simulink model "MMMS_v2_dynamics"  (R2024b)
settings: Solver=VariableStepAuto  StartTime=0.0  StopTime=60  FixedStep=0.001  RelTol=1e-3
InitFcn:
  | %rho_0t=[0.29;0.29;0.29]; %m
  | %V_0t=[-0.001;-0.001;0];%[-0.0005;-0.0005;0];
  | %w_t=[0;0;-0.002];
  | 
  | 
  | %rho_0t=[0.3;0.3;0.2]; %m
  | %V_0t=[-0.001;-0.001;0];%[-0.0005;-0.0005;0];
  | %w_t=[0;0;-0.001];
values from neighbouring files (symbols this model uses):
  Dt = 0.1    [main_EKF.m]
  Fake_Manip_grad = -0.2.*eye(7)    [Initiate_FQ.m]
  g_cm = zeros(4,4,n)    [Initiate_KUKA_inv.m]    (also in Main_MMMS.m; test_KUKA_elements.m)
  g_It00 = [eye(3) rho_It;0 0 0 1]    [main_EKF.m]
  iota0 = eye(6,6)    [Initiate_KUKA_inv.m]    (also in Main_MMMS.m; test_KUKA_elements.m)
  K_d = 10*[1.3*eye(3) zeros(3);zeros(3) 0.8*eye(3)]    [Initiate_FQ.m]    (also in Initiate_KUKA_inv.m = 5*[0.7*eye(3) zeros(3);zeros(3) 0.5*eye(3)]; MMMS_Initiate_FQ.m; Main_MMMS.m = 5*[0.7*eye(3) zeros(3);zeros(3) 0.5*eye(3)]; test_KUKA_elements.m = 50*[0.7*eye(3) zeros(3);zeros(3) 0.5*eye(3)])
  K_i = 5*[0.1*eye(3) zeros(3);zeros(3) 0.01*eye(3)]    [Initiate_FQ.m]    (also in Initiate_KUKA_inv.m = 5*[0.01*eye(3) zeros(3);zeros(3) 0.001*eye(3)]; MMMS_Initiate_FQ.m; Main_MMMS.m = 5*[0.01*eye(3) zeros(3);zeros(3) 0.001*eye(3)]; test_KUKA_elements.m = 50*[0.01*eye(3) zeros(3);zeros(3) 0.001*eye(3)])
  K_p = 100*[0.1 0 0 0 0 0;0 0.1 0 0 0 0; 0 0 0.1 0 0 0; 0 0 0 0.01 0 0 ... (first row only)    [Initiate_FQ.m]    (also in Initiate_KUKA_inv.m = 5*[0.1 0 0 0 0 0;0 0.1 0 0 0 0; 0 0 0.1 0 0 0; 0 0 0 0.01 0 ; MMMS_Initiate_FQ.m; Main_MMMS.m = 5*[0.1 0 0 0 0 0;0 0.1 0 0 0 0; 0 0 0.1 0 0 0; 0 0 0 0.01 0 ; test_KUKA_elements.m = 50*[0.1 0 0 0 0 0;0 0.1 0 0 0 0; 0 0 0.1 0 0 0; 0 0 0 0.01 0)
  K_w = 200*eye(7)    [Initiate_FQ.m]    (also in MMMS_Initiate_FQ.m)
  K_wd = 2*eye(7)    [Initiate_FQ.m]    (also in MMMS_Initiate_FQ.m)
  m = randn(s,total_time_steps,6)*chol(R)    [main_EKF.m]
  M0 = M_temp.M0.data(:,:,1)    [Initiate_FQ.m]    (also in MMMS_Initiate_FQ.m; test_KUKA_elements.m)
  m0 = robot.Bodies{1,n+1}.Mass    [Initiate_KUKA_inv.m]    (also in Main_MMMS.m; test_KUKA_elements.m)
  m0_frak = diag_M(1:6,1:6)    [Initiate_KUKA_inv.m]    (also in Main_MMMS.m; make_uncertain.m = diag_M_unc(1:6,1:6); test_KUKA_elements.m)
  M0m = M_temp.M0m.data(:,:,1)    [Initiate_FQ.m]    (also in MMMS_Initiate_FQ.m; test_KUKA_elements.m)
  m_diag = diag_M(7:end,7:end)    [Initiate_KUKA_inv.m]    (also in Main_MMMS.m; make_uncertain.m = diag_M_unc(7:end,7:end); test_KUKA_elements.m)
  M_t = (((Adjoint(g_It))'\M_t_body)/(Adjoint(g_It)))    [Initiate_FQ.m]    (also in Initiate_KUKA_inv.m = [eye(3)*mt zeros(3); zeros(3) eye(3)*80]; MMMS_Initiate_FQ.m; Main_MMMS.m = [eye(3)*mt zeros(3); zeros(3) eye(3)*80]; test_KUKA_elements.m = [eye(3)*mt zeros(3); zeros(3) eye(3)*80])
  M_t_body = [eye(3)*mt zeros(3); zeros(3) eye(3)*0.416667]    [Initiate_FQ.m]    (also in MMMS_Initiate_FQ.m)
  mm = zeros(1,n)    [Initiate_KUKA_inv.m]    (also in Main_MMMS.m; test_KUKA_elements.m)
  mu = P0    [Initiate_FQ.m]    (also in Initiate_KUKA_inv.m = zeros(6,1); MMMS_Initiate_FQ.m; Main_MMMS.m = zeros(6,1); make_uncertain.m = P0_unc)
  mu_t = inv((Adjoint(g_It))')*M_t_body*[V_It;w_t]    [Initiate_FQ.m]    (also in Initiate_KUKA_inv.m = M_t*[V_0t;w_t]; MMMS_Initiate_FQ.m; Main_MMMS.m = M_t*[V_0t;w_t]; make_uncertain.m = inv((Adjoint(g_It))')*M_t_body_unc*[V_It;w_t])
  noise_st = 0.000005    (= 5e-06)    [main_EKF.m]
  q_dot_m = [0;0;0;0;0;0;0]    [Initiate_FQ.m]    (also in Initiate_KUKA_inv.m; MMMS_Initiate_FQ.m; Main_MMMS.m; test_KUKA_elements.m = [0])
  q_m = [0.2;1.2;0.3;2.5;0.5;1.5;0.6]    [Initiate_FQ.m]    (also in Initiate_KUKA_inv.m = [0;0;0;0;0;0;0]; MMMS_Initiate_FQ.m = [0.2;0.2;0.3;0.5;0.5;0.5;0.6]; Main_MMMS.m = [0;0;0;0;0;0;0]; test_KUKA_elements.m = [0.2;1.2;0.3;1.8;0.5;1.3;0.6])
  rho_It = [0;0;1.7]    [Initiate_FQ.m]    (also in MMMS_Initiate_FQ.m)
  s = RandStream.create('mrg32k3a','NumStreams',1)    [main_EKF.m]
  sc_size = 1    [Initiate_KUKA_inv.m]    (also in Main_MMMS.m; test_KUKA_elements.m)
  V_It = [0.0005;0.0005;0]    [Initiate_FQ.m]    (also in MMMS_Initiate_FQ.m = [0.001;0.001;0])
  Xi_m_matrix = zeros(6*n,n)    [Initiate_KUKA_inv.m]    (also in Main_MMMS.m)
undefined symbols (not defined in the file or in its folder): g_cm0, I0, Im, Mm, X, Xi_m, Y, Z
libraries: nesl_utility x314, sm_lib x231, robotcorelib x30, simulink x12
(part 4 of 14)

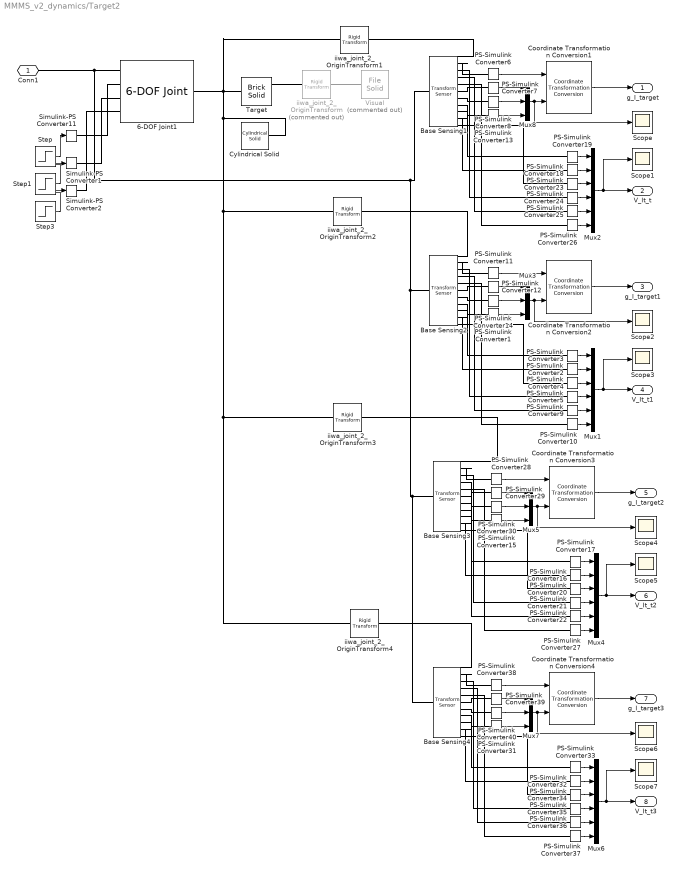
== system MMMS_v2_dynamics/Target2 ==
  6-DOF Joint1 : sm_lib/Joints/6-DOF Joint  JointMode=Normal  CompositeWrenchDir=FollowerOnBase  CompositeWrenchFrame=BaseFrame  SenseConstraintForce=off  SenseConstraintTorque=off  SenseTotalForce=off  SenseTotalTorque=off  PxPositionTargetSpecify=on  PxPositionTargetPriority=High  PxPositionTargetValue=rho_It(1)  PxPositionTargetValueUnits=m  PxVelocityTargetSpecify=on  PxVelocityTargetPriority=High  PxVelocityTargetValue=V_It(1)  PxVelocityTargetValueUnits=m/s  PxEquilibriumPosition=0  PxEquilibriumPositionUnits=m  PxSpringStiffness=0  PxSpringStiffnessUnits=N/m  PxDampingCoefficient=0  PxDampingCoefficientUnits=N/(m/s)  PxLowerLimitSpecify=off  PxLowerLimitBound=-1  PxLowerLimitBoundUnits=m  PxLowerLimitStiffness=1e6  PxLowerLimitStiffnessUnits=N/m  PxLowerLimitDamping=1e3  PxLowerLimitDampingUnits=N/(m/s)  PxLowerLimitTransitionRegionWidth=1e-4  PxLowerLimitTransitionRegionWidthUnits=m  PxUpperLimitSpecify=off  PxUpperLimitBound=1  PxUpperLimitBoundUnits=m  PxUpperLimitStiffness=1e6  PxUpperLimitStiffnessUnits=N/m  PxUpperLimitDamping=1e3  PxUpperLimitDampingUnits=N/(m/s)  PxUpperLimitTransitionRegionWidth=1e-4  PxUpperLimitTransitionRegionWidthUnits=m  PxTorqueActuationMode=InputTorque  PxMotionActuationMode=ComputedMotion  PxSensePosition=off  PxSenseVelocity=off  PxSenseAcceleration=off  PxSenseTorqueForce=off  PxSenseLowerLimitTorqueForce=off  PxSenseUpperLimitTorqueForce=off  PyPositionTargetSpecify=on  PyPositionTargetPriority=High  PyPositionTargetValue=rho_It(2)  PyPositionTargetValueUnits=m  PyVelocityTargetSpecify=on  PyVelocityTargetPriority=High  PyVelocityTargetValue=V_It(2)  PyVelocityTargetValueUnits=m/s  PyEquilibriumPosition=0  PyEquilibriumPositionUnits=m  PySpringStiffness=0  PySpringStiffnessUnits=N/m  PyDampingCoefficient=0  PyDampingCoefficientUnits=N/(m/s)  PyLowerLimitSpecify=off  PyLowerLimitBound=-1  PyLowerLimitBoundUnits=m  PyLowerLimitStiffness=1e6  PyLowerLimitStiffnessUnits=N/m  PyLowerLimitDamping=1e3  PyLowerLimitDampingUnits=N/(m/s)  PyLowerLimitTransitionRegionWidth=1e-4  PyLowerLimitTransitionRegionWidthUnits=m  PyUpperLimitSpecify=off  PyUpperLimitBound=1  PyUpperLimitBoundUnits=m  PyUpperLimitStiffness=1e6  PyUpperLimitStiffnessUnits=N/m  PyUpperLimitDamping=1e3  PyUpperLimitDampingUnits=N/(m/s)  PyUpperLimitTransitionRegionWidth=1e-4  PyUpperLimitTransitionRegionWidthUnits=m  PyTorqueActuationMode=InputTorque  PyMotionActuationMode=ComputedMotion  PySensePosition=off  PySenseVelocity=off  PySenseAcceleration=off  PySenseTorqueForce=off  PySenseLowerLimitTorqueForce=off  PySenseUpperLimitTorqueForce=off  PzPositionTargetSpecify=on  PzPositionTargetPriority=High  PzPositionTargetValue=rho_It(3)-0.1  PzPositionTargetValueUnits=m  PzVelocityTargetSpecify=on  PzVelocityTargetPriority=High  PzVelocityTargetValue=V_It(3)  PzVelocityTargetValueUnits=m/s  PzEquilibriumPosition=0  PzEquilibriumPositionUnits=m  PzSpringStiffness=0  PzSpringStiffnessUnits=N/m  PzDampingCoefficient=0  PzDampingCoefficientUnits=N/(m/s)  PzLowerLimitSpecify=off  PzLowerLimitBound=-1  PzLowerLimitBoundUnits=m  PzLowerLimitStiffness=1e6  PzLowerLimitStiffnessUnits=N/m  PzLowerLimitDamping=1e3  PzLowerLimitDampingUnits=N/(m/s)  PzLowerLimitTransitionRegionWidth=1e-4  PzLowerLimitTransitionRegionWidthUnits=m  PzUpperLimitSpecify=off  PzUpperLimitBound=1  PzUpperLimitBoundUnits=m  PzUpperLimitStiffness=1e6  PzUpperLimitStiffnessUnits=N/m  PzUpperLimitDamping=1e3  PzUpperLimitDampingUnits=N/(m/s)  PzUpperLimitTransitionRegionWidth=1e-4  PzUpperLimitTransitionRegionWidthUnits=m  PzTorqueActuationMode=InputTorque  PzMotionActuationMode=ComputedMotion  PzSensePosition=off  PzSenseVelocity=off  PzSenseAcceleration=off  PzSenseTorqueForce=off  PzSenseLowerLimitTorqueForce=off  PzSenseUpperLimitTorqueForce=off  SphPositionTargetSpecify=on  SphPositionTargetPriority=High  SphPositionTargetRotationMethod=RotationSequence  SphPositionTargetFollAlignAxisA=+X  SphPositionTargetBaseAlignAxisA=+Y  SphPositionTargetFollAlignAxisB=+Y  SphPositionTargetBaseAlignAxisB=+Z  SphPositionTargetRotationStandardAxis=+Z  SphPositionTargetRotationAngle=0.0  SphPositionTargetRotationAngleUnits=deg  SphPositionTargetRotationArbitraryAxis=[0 0 1]  SphPositionTargetRotationSequenceAxes=FollowerAxes  SphPositionTargetRotationSequence=XYZ  SphPositionTargetRotationSequenceAngles=[0 0 0]  SphPositionTargetRotationSequenceAnglesUnits=rad  SphPositionTargetRotationMatrix=[1 0 0; 0 1 0; 0 0 1]  SphPositionTargetQuaternion=[1 0 0 0]  SphVelocityTargetSpecify=on  SphVelocityTargetPriority=High  SphVelocityTargetValue=w_t  SphVelocityTargetValueUnits=rad/s  SphVelocityTargetInFollowerFrame=off  SphEqPosRotationMethod=None  SphEqPosFollAlignAxisA=+X  SphEqPosBaseAlignAxisA=+Y  SphEqPosFollAlignAxisB=+Y  SphEqPosBaseAlignAxisB=+Z  SphEqPosRotationStandardAxis=+Z  SphEqPosRotationAngle=0.0  SphEqPosRotationAngleUnits=deg  SphEqPosRotationArbitraryAxis=[0 0 1]  SphEqPosRotationSequenceAxes=FollowerAxes  SphEqPosRotationSequence=XYX  SphEqPosRotationSequenceAngles=[0 0 0]  SphEqPosRotationSequenceAnglesUnits=deg  SphEqPosRotationMatrix=[1 0 0; 0 1 0; 0 0 1]  SphEqPosQuaternion=[1 0 0 0]  SphSpringStiffness=0  SphSpringStiffnessUnits=N*m/deg  SphDampingCoefficient=0  SphDampingCoefficientUnits=N*m/(deg/s)  SphLowerLimitSpecify=off  SphLowerLimitBound=15  SphLowerLimitBoundUnits=deg  SphLowerLimitStiffness=1e4  SphLowerLimitStiffnessUnits=N*m/deg  SphLowerLimitDamping=10  SphLowerLimitDampingUnits=N*m/(deg/s)  SphLowerLimitTransitionRegionWidth=0.1  SphLowerLimitTransitionRegionWidthUnits=deg  SphUpperLimitSpecify=off  SphUpperLimitBound=45  SphUpperLimitBoundUnits=deg  SphUpperLimitStiffness=1e4  SphUpperLimitStiffnessUnits=N*m/deg  SphUpperLimitDamping=10  SphUpperLimitDampingUnits=N*m/(deg/s)  SphUpperLimitTransitionRegionWidth=0.1  SphUpperLimitTransitionRegionWidthUnits=deg  SphTorqueActuationMode=NoTorque  SphActuateTorqueX=off  SphActuateTorqueY=off  SphActuateTorqueZ=off  SphActuateTorque=off  SphActuationFrame=BaseFrame  SphSensePosition=off  SphSenseVelocityX=off  SphSenseVelocityY=off  SphSenseVelocityZ=off  SphSenseVelocity=off  SphSenseAccelerationX=off  SphSenseAccelerationY=off  SphSenseAccelerationZ=off  SphSenseAcceleration=off  SphSenseLowerLimitTorqueMag=off  SphSenseUpperLimitTorqueMag=off  SphSensingFrame=BaseFrame
  Base Sensing{1..4} (4 alike) : sm_lib/Frames and Transforms/Transform Sensor  MeasurementFrame=NonRotatingBase  RotationSequence=XYZ  SenseAngle=off  SenseAxis=off  SenseQ=off  SenseR=on  SenseRotationSequence=off  SenseOmegaX=on  SenseOmegaY=on  SenseOmegaZ=on  SenseOmega=off  SenseQDot=off  SenseRDot=off  SenseRotationSequenceDot=off  SenseAlphaX=off  SenseAlphaY=off  SenseAlphaZ=off  SenseAlpha=off  SenseQDDot=off  SenseRDDot=off  SenseX=on  SenseY=on  SenseZ=on  SenseXYZ=off  SenseRad=off  SenseAzim=off  SenseDist=off  SenseInc=off  SenseXDot=on  SenseYDot=on  SenseZDot=on  SenseXYZDot=off  SenseRadDot=off  SenseAzimDot=off  SenseDistDot=off  SenseIncDot=off  SenseXDDot=off  SenseYDDot=off  SenseZDDot=off  SenseXYZDDot=off  SenseRadDDot=off  SenseAzimDDot=off  SenseDistDDot=off  SenseIncDDot=off
  Coordinate Transformation Conversion{1..4} (4 alike) : robotcorelib/Coordinate Transformation Conversion  InputRepresentation=Rotation Matrix  InputEulerSequence=ZYX  ShowTrVecInputPort=on  OutputRepresentation=Homogeneous Transformation  OutputEulerSequence=ZYX  ShowTrVecOutputPort=on  SimulateUsing=Interpreted execution
  Cylindrical Solid : sm_lib/Body Elements/Cylindrical Solid  CylinderRadius=1  CylinderRadiusUnits=m  CylinderLength=0.001  CylinderLengthUnits=m  ExportEntireGeometry=off  InertiaType=CalculateFromGeometry  BasedOnType=Density  Density=0  DensityUnits=kg/m^3  Mass=1  MassUnits=kg  CenterOfMass=[0 0 0]  CenterOfMassUnits=m  MomentsOfInertia=[1 1 1]  MomentsOfInertiaUnits=kg*m^2  ProductsOfInertia=[0 0 0]  ProductsOfInertiaUnits=kg*m^2  GraphicType=FromGeometry  MarkerShape=Sphere  MarkerSize=10  GraphicVisPropType=SimpleVisualProperties  GraphicDiffuseColor=[1.0 0.0 0.0]  GraphicOpacity=0.4  GraphicSpecularColor=[0.5 0.5 0.5 1.0]  GraphicAmbientColor=[0.15 0.15 0.15 1.0]  GraphicEmissiveColor=[0.0 0.0 0.0 1.0]  GraphicShininess=75  DoExposeReferenceFrame=on  SerializedFrames=<Frames/>
  Mux{1..2,4,6} (4 alike) : Mux  Inputs=6
  Mux{3,5,7..8} (4 alike) : Mux  Inputs=3
  PS-Simulink Converter{1..40} (40 alike) : nesl_utility/PS-Simulink Converter  PhysicalDomain=network_engine_domain  SubClassName=ps_output  LeftPortType=input  RightPortType=output  PseudoPeriodic=off  Frequencies=[]  VectorFormat=1-D array  Unit=inherit  AffineConversion=off
  Scope{,1..7} (8 alike) : Scope
  Simulink-PS Converter1 : nesl_utility/Simulink-PS Converter  PhysicalDomain=network_engine_domain  SubClassName=ps_input  LeftPortType=input  RightPortType=output  PseudoPeriodic=off  Frequencies=[]  NoiseDistribution=none  NoiseParameters=[]  Unit=1  AffineConversion=off  FilteringAndDerivatives=provide  SimscapeFilterOrder=1  InputFilterTimeConstant=0.001  UdotUserProvided=0
  Simulink-PS Converter11 : nesl_utility/Simulink-PS Converter  PhysicalDomain=network_engine_domain  SubClassName=ps_input  LeftPortType=input  RightPortType=output  PseudoPeriodic=off  Frequencies=[]  NoiseDistribution=none  NoiseParameters=[]  Unit=1  AffineConversion=off  FilteringAndDerivatives=provide  SimscapeFilterOrder=1  InputFilterTimeConstant=0.001  UdotUserProvided=0
  Simulink-PS Converter2 : nesl_utility/Simulink-PS Converter  PhysicalDomain=network_engine_domain  SubClassName=ps_input  LeftPortType=input  RightPortType=output  PseudoPeriodic=off  Frequencies=[]  NoiseDistribution=none  NoiseParameters=[]  Unit=1  AffineConversion=off  FilteringAndDerivatives=provide  SimscapeFilterOrder=1  InputFilterTimeConstant=0.001  UdotUserProvided=0
  Step : Step  Time=50  After=-0.004  SampleTime=0
  Step1 : Step  Time=50  After=-0.004  SampleTime=0
  Step3 : Step  Time=50  After=-0.0002  SampleTime=0
  Target : sm_lib/Body Elements/Brick Solid  BrickDimensions=[0.5, 0.5, 0.5]  BrickDimensionsUnits=m  ExportEntireGeometry=on  InertiaType=Custom  BasedOnType=Mass  Density=1000  DensityUnits=kg/m^3  Mass=10  MassUnits=kg  CenterOfMass=[0 0 0]  CenterOfMassUnits=m  MomentsOfInertia=[M_t(4,4) M_t(5,5) M_t(6,6)]  MomentsOfInertiaUnits=kg*m^2  ProductsOfInertia=[0 0 0]  ProductsOfInertiaUnits=kg*m^2  GraphicType=None  MarkerShape=Sphere  MarkerSize=10  GraphicVisPropType=SimpleVisualProperties  GraphicDiffuseColor=[1.0 0.0 0.0]  GraphicOpacity=1.0  GraphicSpecularColor=[0.5 0.5 0.5 1.0]  GraphicAmbientColor=[0.15 0.15 0.15 1.0]  GraphicEmissiveColor=[0.0 0.0 0.0 1.0]  GraphicShininess=75  DoExposeReferenceFrame=on  SerializedFrames=<Frames><Frame><Id>Frame1</Id><Value><Name>F1</Name><Origin><Source>GeometricFeature</Source><FeatureName>-x -y -z point</FeatureName></Origin><PrimaryAxis><DefinedDirection>+Z</DefinedDirection><Source>ReferenceFrame</Source><SourceDirection>+Z</SourceDirection><FeatureName></FeatureName></PrimaryAxis><SecondaryAxis><DefinedDirection>+X</DefinedDirection><Source>ReferenceFrame</Source><SourceDirection>+X</SourceDirection><FeatureName></FeatureName></SecondaryAxis></Value></Frame></Frames>
  Visual : sm_lib/Body Elements/File Solid  Commented=on  ExtGeomFileName=Spacecrafts/CubeSatAssembly_wo_antennas.stl  UnitType=Custom  ExtGeomFileUnits=cm  StepReaderType=HEX  ExportConvexHullGeometry=off  InertiaType=Custom  BasedOnType=DensityFromFile  Density=1000  DensityUnits=kg/m^3  Mass=0  MassUnits=kg  CenterOfMass=[0, 0, 0]  CenterOfMassUnits=m  MomentsOfInertia=[0, 0, 0]  MomentsOfInertiaUnits=kg*m^2  ProductsOfInertia=[0, 0, 0]  ProductsOfInertiaUnits=kg*m^2  GraphicType=FromGeometry  MarkerShape=Sphere  MarkerSize=10  GraphicVisPropType=SimpleVisualProperties  GraphicDiffuseColor=[0.7 0.7 0.7]  GraphicOpacity=1  GraphicSpecularColor=[0.5 0.5 0.5 1.0]  GraphicAmbientColor=[0.15 0.15 0.15 1.0]  GraphicEmissiveColor=[0.0 0.0 0.0 1.0]  GraphicShininess=75  DoExposeReferenceFrame=on  SerializedFrames=<Frames/>
  iiwa_joint_2_OriginTransform : sm_lib/Frames and Transforms/Rigid Transform  Commented=on  RotationMethod=RotationSequence  FollAlignAxisA=+X  BaseAlignAxisA=+Y  FollAlignAxisB=+Y  BaseAlignAxisB=+Z  RotationStandardAxis=+Z  RotationAngle=0.0  RotationAngleUnits=deg  RotationArbitraryAxis=[0 0 1]  RotationSequenceAxes=FollowerAxes  RotationSequence=XYZ  RotationSequenceAngles=[0 0 0]  RotationSequenceAnglesUnits=rad  RotationMatrix=[1 0 0; 0 1 0; 0 0 1]  Quaternion=[1 0 0 0]  TranslationMethod=Cartesian  TranslationCartesianOffset=[-3.28, -4.43, 0.817]+[0.25, 0.25, 0.25]  TranslationCartesianOffsetUnits=m  TranslationStandardAxis=+Z  TranslationStandardOffset=0  TranslationStandardOffsetUnits=m  TranslationROffset=0  TranslationROffsetUnits=m  TranslationThetaOffset=0  TranslationThetaOffsetUnits=deg  TranslationZOffset=0  TranslationZOffsetUnits=m
  iiwa_joint_2_OriginTransform1 : sm_lib/Frames and Transforms/Rigid Transform  RotationMethod=RotationSequence  FollAlignAxisA=+X  BaseAlignAxisA=+Y  FollAlignAxisB=+Y  BaseAlignAxisB=+Z  RotationStandardAxis=+Z  RotationAngle=0.0  RotationAngleUnits=deg  RotationArbitraryAxis=[0 0 1]  RotationSequenceAxes=FollowerAxes  RotationSequence=XYZ  RotationSequenceAngles=[0 0 0]  RotationSequenceAnglesUnits=rad  RotationMatrix=[1 0 0; 0 1 0; 0 0 1]  Quaternion=[1 0 0 0]  TranslationMethod=Cartesian  TranslationCartesianOffset=[-1,0,0]  TranslationCartesianOffsetUnits=m  TranslationStandardAxis=+Z  TranslationStandardOffset=0  TranslationStandardOffsetUnits=m  TranslationROffset=0  TranslationROffsetUnits=m  TranslationThetaOffset=0  TranslationThetaOffsetUnits=deg  TranslationZOffset=0  TranslationZOffsetUnits=m
  iiwa_joint_2_OriginTransform2 : sm_lib/Frames and Transforms/Rigid Transform  RotationMethod=RotationSequence  FollAlignAxisA=+X  BaseAlignAxisA=+Y  FollAlignAxisB=+Y  BaseAlignAxisB=+Z  RotationStandardAxis=+Z  RotationAngle=0.0  RotationAngleUnits=deg  RotationArbitraryAxis=[0 0 1]  RotationSequenceAxes=FollowerAxes  RotationSequence=XYZ  RotationSequenceAngles=[0 0 0]  RotationSequenceAnglesUnits=rad  RotationMatrix=[1 0 0; 0 1 0; 0 0 1]  Quaternion=[1 0 0 0]  TranslationMethod=Cartesian  TranslationCartesianOffset=[sqrt(0.5),sqrt(0.5),0]  TranslationCartesianOffsetUnits=m  TranslationStandardAxis=+Z  TranslationStandardOffset=0  TranslationStandardOffsetUnits=m  TranslationROffset=0  TranslationROffsetUnits=m  TranslationThetaOffset=0  TranslationThetaOffsetUnits=deg  TranslationZOffset=0  TranslationZOffsetUnits=m
  iiwa_joint_2_OriginTransform3 : sm_lib/Frames and Transforms/Rigid Transform  RotationMethod=RotationSequence  FollAlignAxisA=+X  BaseAlignAxisA=+Y  FollAlignAxisB=+Y  BaseAlignAxisB=+Z  RotationStandardAxis=+Z  RotationAngle=0.0  RotationAngleUnits=deg  RotationArbitraryAxis=[0 0 1]  RotationSequenceAxes=FollowerAxes  RotationSequence=XYZ  RotationSequenceAngles=[0 0 0]  RotationSequenceAnglesUnits=rad  RotationMatrix=[1 0 0; 0 1 0; 0 0 1]  Quaternion=[1 0 0 0]  TranslationMethod=Cartesian  TranslationCartesianOffset=[sqrt(0.5),-sqrt(0.5),0]  TranslationCartesianOffsetUnits=m  TranslationStandardAxis=+Z  TranslationStandardOffset=0  TranslationStandardOffsetUnits=m  TranslationROffset=0  TranslationROffsetUnits=m  TranslationThetaOffset=0  TranslationThetaOffsetUnits=deg  TranslationZOffset=0  TranslationZOffsetUnits=m
  iiwa_joint_2_OriginTransform4 : sm_lib/Frames and Transforms/Rigid Transform  RotationMethod=RotationSequence  FollAlignAxisA=+X  BaseAlignAxisA=+Y  FollAlignAxisB=+Y  BaseAlignAxisB=+Z  RotationStandardAxis=+Z  RotationAngle=0.0  RotationAngleUnits=deg  RotationArbitraryAxis=[0 0 1]  RotationSequenceAxes=FollowerAxes  RotationSequence=XYZ  RotationSequenceAngles=[0 0 0]  RotationSequenceAnglesUnits=rad  RotationMatrix=[1 0 0; 0 1 0; 0 0 1]  Quaternion=[1 0 0 0]  TranslationMethod=Cartesian  TranslationCartesianOffset=[0,1,0]  TranslationCartesianOffsetUnits=m  TranslationStandardAxis=+Z  TranslationStandardOffset=0  TranslationStandardOffsetUnits=m  TranslationROffset=0  TranslationROffsetUnits=m  TranslationThetaOffset=0  TranslationThetaOffsetUnits=deg  TranslationZOffset=0  TranslationZOffsetUnits=m
  Conn1 : PMIOPort  Side=Left
  g_I_target : Outport
  V_It_t : Outport  Port=2
  g_I_target1 : Outport  Port=3
  V_It_t1 : Outport  Port=4
  g_I_target2 : Outport  Port=5
  V_It_t2 : Outport  Port=6
  g_I_target3 : Outport  Port=7
  V_It_t3 : Outport  Port=8
  wires:
  PS-Simulink Converter13/1 -> Mux8/3
  Coordinate Transformation Conversion1/1 -> g_I_target/1
  PS-Simulink Converter7/1 -> Mux8/1
  PS-Simulink Converter6/1 -> Coordinate Transformation Conversion1/1
  PS-Simulink Converter8/1 -> Mux8/2
  Mux8/1 -> Scope/1, Coordinate Transformation Conversion1/2
  PS-Simulink Converter24/1 -> Mux2/4
  PS-Simulink Converter18/1 -> Mux2/2
  PS-Simulink Converter25/1 -> Mux2/5
  Mux2/1 -> Scope1/1, V_It_t/1
  PS-Simulink Converter19/1 -> Mux2/1
  PS-Simulink Converter23/1 -> Mux2/3
  PS-Simulink Converter26/1 -> Mux2/6
  Step/1 -> Simulink-PS Converter11/1
  Step1/1 -> Simulink-PS Converter1/1
  Step3/1 -> Simulink-PS Converter2/1
  PS-Simulink Converter4/1 -> Mux1/3
  PS-Simulink Converter5/1 -> Mux1/4
  PS-Simulink Converter2/1 -> Mux1/2
  PS-Simulink Converter3/1 -> Mux1/1
  PS-Simulink Converter9/1 -> Mux1/5
  PS-Simulink Converter10/1 -> Mux1/6
  PS-Simulink Converter1/1 -> Mux3/3
  Coordinate Transformation Conversion2/1 -> g_I_target1/1
  PS-Simulink Converter11/1 -> Coordinate Transformation Conversion2/1
  PS-Simulink Converter14/1 -> Mux3/2
  Mux3/1 -> Scope2/1, Coordinate Transformation Conversion2/2
  PS-Simulink Converter12/1 -> Mux3/1
  Mux1/1 -> Scope3/1, V_It_t1/1
  PS-Simulink Converter20/1 -> Mux4/3
  PS-Simulink Converter21/1 -> Mux4/4
  PS-Simulink Converter16/1 -> Mux4/2
  PS-Simulink Converter17/1 -> Mux4/1
  PS-Simulink Converter22/1 -> Mux4/5
  PS-Simulink Converter27/1 -> Mux4/6
  PS-Simulink Converter15/1 -> Mux5/3
  Coordinate Transformation Conversion3/1 -> g_I_target2/1
  PS-Simulink Converter28/1 -> Coordinate Transformation Conversion3/1
  PS-Simulink Converter30/1 -> Mux5/2
  Mux5/1 -> Scope4/1, Coordinate Transformation Conversion3/2
  PS-Simulink Converter29/1 -> Mux5/1
  Mux4/1 -> Scope5/1, V_It_t2/1
  PS-Simulink Converter34/1 -> Mux6/3
  PS-Simulink Converter35/1 -> Mux6/4
  PS-Simulink Converter32/1 -> Mux6/2
  PS-Simulink Converter33/1 -> Mux6/1
  PS-Simulink Converter36/1 -> Mux6/5
  PS-Simulink Converter37/1 -> Mux6/6
  PS-Simulink Converter31/1 -> Mux7/3
  Coordinate Transformation Conversion4/1 -> g_I_target3/1
  PS-Simulink Converter38/1 -> Coordinate Transformation Conversion4/1
  PS-Simulink Converter40/1 -> Mux7/2
  Mux7/1 -> Scope6/1, Coordinate Transformation Conversion4/2
  PS-Simulink Converter39/1 -> Mux7/1
  Mux6/1 -> Scope7/1, V_It_t3/1
  connections:
  Target/RConn1 -- iiwa_joint_2_OriginTransform4/LConn1 -- iiwa_joint_2_OriginTransform3/LConn1 -- iiwa_joint_2_OriginTransform2/LConn1 -- Cylindrical Solid/RConn1 -- iiwa_joint_2_OriginTransform1/LConn1 -- 6-DOF Joint1/RConn1
  Base Sensing1/RConn2 -- PS-Simulink Converter6/LConn1
  Base Sensing1/RConn3 -- PS-Simulink Converter24/LConn1
  Base Sensing1/LConn1 -- Conn1/RConn1 -- 6-DOF Joint1/LConn1 -- Base Sensing4/LConn1 -- Base Sensing3/LConn1 -- Base Sensing2/LConn1
  Base Sensing1/RConn5 -- PS-Simulink Converter26/LConn1
  Visual/RConn1 -- iiwa_joint_2_OriginTransform/RConn1
  Base Sensing1/RConn4 -- PS-Simulink Converter25/LConn1
  Base Sensing1/RConn6 -- PS-Simulink Converter7/LConn1
  Base Sensing1/RConn7 -- PS-Simulink Converter8/LConn1
  Base Sensing1/RConn8 -- PS-Simulink Converter13/LConn1
  Base Sensing1/RConn9 -- PS-Simulink Converter19/LConn1
  Base Sensing1/RConn10 -- PS-Simulink Converter18/LConn1
  Base Sensing1/RConn11 -- PS-Simulink Converter23/LConn1
  Target/LConn1 -- iiwa_joint_2_OriginTransform/LConn1
  6-DOF Joint1/LConn2 -- Simulink-PS Converter11/RConn1
  6-DOF Joint1/LConn3 -- Simulink-PS Converter1/RConn1
  Simulink-PS Converter2/RConn1 -- 6-DOF Joint1/LConn4
  Base Sensing2/RConn3 -- PS-Simulink Converter5/LConn1
  Base Sensing2/RConn10 -- PS-Simulink Converter2/LConn1
  Base Sensing2/RConn2 -- PS-Simulink Converter11/LConn1
  Base Sensing2/RConn7 -- PS-Simulink Converter14/LConn1
  Base Sensing2/RConn6 -- PS-Simulink Converter12/LConn1
  Base Sensing2/RConn8 -- PS-Simulink Converter1/LConn1
  Base Sensing2/RConn5 -- PS-Simulink Converter10/LConn1
  Base Sensing2/RConn9 -- PS-Simulink Converter3/LConn1
  Base Sensing2/RConn11 -- PS-Simulink Converter4/LConn1
  Base Sensing2/RConn4 -- PS-Simulink Converter9/LConn1
  Base Sensing3/RConn3 -- PS-Simulink Converter21/LConn1
  Base Sensing3/RConn10 -- PS-Simulink Converter16/LConn1
  Base Sensing3/RConn2 -- PS-Simulink Converter28/LConn1
  Base Sensing3/RConn7 -- PS-Simulink Converter30/LConn1
  Base Sensing3/RConn6 -- PS-Simulink Converter29/LConn1
  Base Sensing3/RConn8 -- PS-Simulink Converter15/LConn1
  Base Sensing3/RConn5 -- PS-Simulink Converter27/LConn1
  Base Sensing3/RConn9 -- PS-Simulink Converter17/LConn1
  Base Sensing3/RConn11 -- PS-Simulink Converter20/LConn1
  Base Sensing3/RConn4 -- PS-Simulink Converter22/LConn1
  Base Sensing4/RConn3 -- PS-Simulink Converter35/LConn1
  Base Sensing4/RConn10 -- PS-Simulink Converter32/LConn1
  Base Sensing4/RConn2 -- PS-Simulink Converter38/LConn1
  Base Sensing4/RConn7 -- PS-Simulink Converter40/LConn1
  Base Sensing4/RConn6 -- PS-Simulink Converter39/LConn1
  Base Sensing4/RConn8 -- PS-Simulink Converter31/LConn1
  Base Sensing4/RConn5 -- PS-Simulink Converter37/LConn1
  Base Sensing4/RConn9 -- PS-Simulink Converter33/LConn1
  Base Sensing4/RConn11 -- PS-Simulink Converter34/LConn1
  Base Sensing4/RConn4 -- PS-Simulink Converter36/LConn1
  Base Sensing1/RConn1 -- iiwa_joint_2_OriginTransform1/RConn1
  iiwa_joint_2_OriginTransform2/RConn1 -- Base Sensing2/RConn1
  Base Sensing3/RConn1 -- iiwa_joint_2_OriginTransform3/RConn1
  iiwa_joint_2_OriginTransform4/RConn1 -- Base Sensing4/RConn1

== system MMMS_v2_dynamics/Controller1/Kinematics ==
  g_I0 : Inport
  g_It : Inport  Port=2
  V_It : Inport  Port=3
  Divide : Product  Inputs=/*  Multiplication=Matrix(*)
  E_g : Scope
  MATLAB Function : MATLAB Function  TreatAsAtomicUnit=on
  Pose Error Function : MATLAB Function  TreatAsAtomicUnit=on
  Scope : Scope
  Scope2 : Scope
  Scope3 : Scope
  Subtract : Sum  Inputs=+-
  Terminator3 : Terminator
  V_It_1 : MATLAB Function  TreatAsAtomicUnit=on
  Velocity_error : MATLAB Function  TreatAsAtomicUnit=on
  g_te1 : Outport
  V_te : Outport  Port=2
  tag scope: E_g_plot=global, g_te=global, v_error_plot=global
  wires:
  g_It/1 -> Velocity_error/4(g_It), Divide/1
  g_I0/1 -> MATLAB Function/1(g_I0), V_It_1/2(g_I0), Scope3/1, Velocity_error/1(g_I0), Divide/2
  Divide/1 -> g_te1/1, [g_te], Pose Error Function/1(g_te)
  Velocity_error/1(V_e) -> V_te/1
  V_It/1 -> Velocity_error/3(V_It), Scope2/1
  [V_Ie] -> MATLAB Function/2(V_Ie_e), Velocity_error/2(V_Ie)
  Pose Error Function/1(E_g) -> E_g/1, [E_g_plot], Terminator3/1
  [V_I0] -> V_It_1/1(V_I0)
  Subtract/1 -> Scope/1
  MATLAB Function/1(V_Ie) -> Subtract/1
  V_It_1/1(V_I0_3) -> Subtract/2
  Velocity_error/2(normV) -> [v_error_plot]

== system MMMS_v2_dynamics/Controller13/Kinematics ==
  g_I0 : Inport
  g_It : Inport  Port=2
  V_It : Inport  Port=3
  Divide : Product  Inputs=/*  Multiplication=Matrix(*)
  E_g : Scope
  Pose Error Function : MATLAB Function  TreatAsAtomicUnit=on
  Scope2 : Scope
  Scope3 : Scope
  Terminator3 : Terminator
  Velocity_error : MATLAB Function  TreatAsAtomicUnit=on
  g_te1 : Outport
  V_te : Outport  Port=2
  tag scope: E_g_plot=global, g_te=global, v_error_plot=global
  wires:
  g_It/1 -> Velocity_error/4(g_It), Divide/1
  g_I0/1 -> Scope3/1, Velocity_error/1(g_I0), Divide/2
  Divide/1 -> g_te1/1, [g_te], Pose Error Function/1(g_te)
  Velocity_error/1(V_e) -> V_te/1
  V_It/1 -> Velocity_error/3(V_It), Scope2/1
  [V_I0] -> Velocity_error/2(V_Ie)
  Pose Error Function/1(E_g) -> E_g/1, [E_g_plot], Terminator3/1
  Velocity_error/2(normV) -> [v_error_plot]

== system MMMS_v2_dynamics/Controller2/Kinematics ==
  g_I0 : Inport
  g_It : Inport  Port=2
  V_It : Inport  Port=3
  Divide : Product  Inputs=/*  Multiplication=Matrix(*)
  E_g : Scope
  MATLAB Function : MATLAB Function  TreatAsAtomicUnit=on
  Pose Error Function : MATLAB Function  TreatAsAtomicUnit=on
  Scope : Scope
  Scope2 : Scope
  Scope3 : Scope
  Subtract : Sum  Inputs=+-
  Terminator3 : Terminator
  V_It_1 : MATLAB Function  TreatAsAtomicUnit=on
  Velocity_error : MATLAB Function  TreatAsAtomicUnit=on
  g_te1 : Outport
  V_te : Outport  Port=2
  tag scope: E_g_plot2=global, g_te2=global, v_error_plot2=global
  wires:
  Velocity_error/2(normV) -> [v_error_plot2]
  V_It_1/1(V_I0_3) -> Subtract/2
  MATLAB Function/1(V_Ie) -> Subtract/1
  Subtract/1 -> Scope/1
  [V_I02] -> V_It_1/1(V_I0)
  Pose Error Function/1(E_g) -> Terminator3/1, [E_g_plot2], E_g/1
  [V_Ie2] -> Velocity_error/2(V_Ie), MATLAB Function/2(V_Ie_e)
  V_It/1 -> Scope2/1, Velocity_error/3(V_It)
  Velocity_error/1(V_e) -> V_te/1
  Divide/1 -> Pose Error Function/1(g_te), [g_te2], g_te1/1
  g_I0/1 -> Divide/2, Velocity_error/1(g_I0), Scope3/1, V_It_1/2(g_I0), MATLAB Function/1(g_I0)
  g_It/1 -> Divide/1, Velocity_error/4(g_It)

== system MMMS_v2_dynamics/Controller23/Filter ==
  z : Inport
  z_gt : Inport  Port=2
  Pulse Generator : DiscretePulseGenerator  PulseType=Time based  Period=Dt  PulseWidth=10
  Scope{17,19..20,22} (4 alike) : Scope
  Scope21 : Scope  NumInputPorts=2
  Transport Delay1 : TransportDelay  DelayTime=Dt  InitialOutput=g_It00  TransDelayFeedthrough=on
  Transport Delay2 : TransportDelay  DelayTime=Dt  InitialOutput=zeros(6)  TransDelayFeedthrough=on
  Triggered Subsystem : Subsystem  TreatAsAtomicUnit=on
  Zero-Order Hold1 : ZeroOrderHold  SampleTime=Dt
  sensing noise in g_t1 : MATLAB Function  TreatAsAtomicUnit=on
  sensing noise in g_t2 : MATLAB Function  TreatAsAtomicUnit=on
  z1 : Outport
  wires:
  sensing noise in g_t2/1(errM) -> Scope21/1  "Measured \\Nabla E_g"
  Transport Delay2/1 -> Triggered Subsystem/2(P_pos)
  Triggered Subsystem/1(X_pos_out) -> Scope17/1, Transport Delay1/1
  z_gt/1 -> sensing noise in g_t1/2(z_gt), sensing noise in g_t2/2(z_gt)
  sensing noise in g_t1/1(errM) -> Scope21/2, Scope20/1  "Filtered \\Nabla E_g"
  Transport Delay1/1 -> Zero-Order Hold1/1, Triggered Subsystem/1(X_pos)
  Pulse Generator/1 -> Triggered Subsystem/Trigger, Scope22/1
  Zero-Order Hold1/1 -> sensing noise in g_t2/1(z), z1/1
  Triggered Subsystem/2(P_pos_out) -> Transport Delay2/1
  z/1 -> Scope19/1, sensing noise in g_t1/1(z), Triggered Subsystem/3(Z)

== system MMMS_v2_dynamics/Controller23/Kinematics ==
  g_I0 : Inport
  g_It : Inport  Port=2
  V_It : Inport  Port=3
  Divide : Product  Inputs=/*  Multiplication=Matrix(*)
  E_g : Scope
  MATLAB Function : MATLAB Function  TreatAsAtomicUnit=on
  Pose Error Function : MATLAB Function  TreatAsAtomicUnit=on
  Scope : Scope
  Scope2 : Scope
  Scope3 : Scope
  Subtract : Sum  Inputs=+-
  Terminator3 : Terminator
  V_It_1 : MATLAB Function  TreatAsAtomicUnit=on
  Velocity_error : MATLAB Function  TreatAsAtomicUnit=on
  g_te1 : Outport
  V_te : Outport  Port=2
  tag scope: E_g_plot=global, g_te=global, v_error_plot=global
  wires:
  g_It/1 -> Velocity_error/4(g_It), Divide/1
  g_I0/1 -> MATLAB Function/1(g_I0), V_It_1/2(g_I0), Scope3/1, Velocity_error/1(g_I0), Divide/2
  Divide/1 -> g_te1/1, [g_te], Pose Error Function/1(g_te)
  Velocity_error/1(V_e) -> V_te/1
  V_It/1 -> Velocity_error/3(V_It), Scope2/1
  [V_Ie] -> MATLAB Function/2(V_Ie_e), Velocity_error/2(V_Ie)
  Pose Error Function/1(E_g) -> E_g/1, [E_g_plot], Terminator3/1
  [V_I0] -> V_It_1/1(V_I0)
  Subtract/1 -> Scope/1
  MATLAB Function/1(V_Ie) -> Subtract/1
  V_It_1/1(V_I0_3) -> Subtract/2
  Velocity_error/2(normV) -> [v_error_plot]

== system MMMS_v2_dynamics/Controller3/Kinematics ==
  g_I0 : Inport
  g_It : Inport  Port=2
  V_It : Inport  Port=3
  Divide : Product  Inputs=/*  Multiplication=Matrix(*)
  E_g : Scope
  MATLAB Function : MATLAB Function  TreatAsAtomicUnit=on
  Pose Error Function : MATLAB Function  TreatAsAtomicUnit=on
  Scope : Scope
  Scope2 : Scope
  Scope3 : Scope
  Subtract : Sum  Inputs=+-
  Terminator3 : Terminator
  V_It_1 : MATLAB Function  TreatAsAtomicUnit=on
  Velocity_error : MATLAB Function  TreatAsAtomicUnit=on
  g_te1 : Outport
  V_te : Outport  Port=2
  tag scope: E_g_plot3=global, g_te3=global, v_error_plot3=global
  wires:
  g_It/1 -> Velocity_error/4(g_It), Divide/1
  g_I0/1 -> MATLAB Function/1(g_I0), V_It_1/2(g_I0), Scope3/1, Velocity_error/1(g_I0), Divide/2
  Divide/1 -> g_te1/1, [g_te3], Pose Error Function/1(g_te)
  Velocity_error/1(V_e) -> V_te/1
  V_It/1 -> Velocity_error/3(V_It), Scope2/1
  [V_Ie3] -> MATLAB Function/2(V_Ie_e), Velocity_error/2(V_Ie)
  Pose Error Function/1(E_g) -> E_g/1, [E_g_plot3], Terminator3/1
  [V_I03] -> V_It_1/1(V_I0)
  Subtract/1 -> Scope/1
  MATLAB Function/1(V_Ie) -> Subtract/1
  V_It_1/1(V_I0_3) -> Subtract/2
  Velocity_error/2(normV) -> [v_error_plot3]

== system MMMS_v2_dynamics/Dynamic Parameters/A_connection1 ==
  M0 : Inport
  M0m : Inport  Port=2
  Divide : Product  Inputs=/*  Multiplication=Matrix(*)
  A : Outport
  wires:
  Divide/1 -> A/1
  M0/1 -> Divide/1
  M0m/1 -> Divide/2

== system MMMS_v2_dynamics/Dynamic Parameters/Mass Matrix Blocks1 ==
  Lm : Inport
  Lm0 : Inport  Port=2
  Xi_m_matrix : Inport  Port=3
  Add : Sum
  Constant1 : Constant  Value=m0_frak  VectorParams1D=off
  Constant2 : Constant  Value=m_diag  VectorParams1D=off
  Matrix Multiply1 : Product  Inputs=4  Multiplication=Matrix(*)
  Matrix Multiply3 : Product  Inputs=5  Multiplication=Matrix(*)
  Matrix Multiply4 : Product  Inputs=3  Multiplication=Matrix(*)
  Matrix Multiply5 : Product  Inputs=1  Multiplication=Matrix(*)
  Transpose3 : Math  Operator=transpose
  Transpose4 : Math  Operator=transpose
  Transpose5 : Math  Operator=transpose
  M0 : Outport
  M0m : Outport  Port=2
  Mm : Outport  Port=3
  tag scope: diag_Mm=global
  wires:
  Xi_m_matrix/1 -> Matrix Multiply1/4, Matrix Multiply3/5, Transpose3/1
  Matrix Multiply5/1 -> M0/1
  Lm0/1 -> Transpose5/1, Matrix Multiply4/3
  Transpose5/1 -> Matrix Multiply4/1, Matrix Multiply1/1
  Transpose4/1 -> Matrix Multiply3/2
  Matrix Multiply3/1 -> Mm/1
  Matrix Multiply1/1 -> M0m/1
  Matrix Multiply4/1 -> Add/2
  Transpose3/1 -> Matrix Multiply3/1
  Lm/1 -> Matrix Multiply1/3, Matrix Multiply3/4, Transpose4/1
  Add/1 -> Matrix Multiply5/1
  Constant2/1 -> Matrix Multiply4/2, Matrix Multiply3/3, Matrix Multiply1/2, [diag_Mm]
  Constant1/1 -> Add/1

== system MMMS_v2_dynamics/Dynamic Parameters1/A_connection1 ==
  M0 : Inport
  M0m : Inport  Port=2
  Divide : Product  Inputs=/*  Multiplication=Matrix(*)
  A : Outport
  wires:
  M0m/1 -> Divide/2
  M0/1 -> Divide/1
  Divide/1 -> A/1

== system MMMS_v2_dynamics/Dynamic Parameters1/Mass Matrix Blocks1 ==
  Lm : Inport
  Lm0 : Inport  Port=2
  Xi_m_matrix : Inport  Port=3
  Add : Sum
  Constant1 : Constant  Value=m0_frak  VectorParams1D=off
  Constant2 : Constant  Value=m_diag  VectorParams1D=off
  Matrix Multiply1 : Product  Inputs=4  Multiplication=Matrix(*)
  Matrix Multiply3 : Product  Inputs=5  Multiplication=Matrix(*)
  Matrix Multiply4 : Product  Inputs=3  Multiplication=Matrix(*)
  Matrix Multiply5 : Product  Inputs=1  Multiplication=Matrix(*)
  Transpose3 : Math  Operator=transpose
  Transpose4 : Math  Operator=transpose
  Transpose5 : Math  Operator=transpose
  M0 : Outport
  M0m : Outport  Port=2
  Mm : Outport  Port=3
  wires:
  Constant1/1 -> Add/1
  Constant2/1 -> Matrix Multiply1/2, Matrix Multiply3/3, Matrix Multiply4/2
  Add/1 -> Matrix Multiply5/1
  Lm/1 -> Transpose4/1, Matrix Multiply3/4, Matrix Multiply1/3
  Transpose3/1 -> Matrix Multiply3/1
  Matrix Multiply4/1 -> Add/2
  Matrix Multiply1/1 -> M0m/1
  Matrix Multiply3/1 -> Mm/1
  Transpose4/1 -> Matrix Multiply3/2
  Transpose5/1 -> Matrix Multiply1/1, Matrix Multiply4/1
  Lm0/1 -> Matrix Multiply4/3, Transpose5/1
  Matrix Multiply5/1 -> M0/1
  Xi_m_matrix/1 -> Transpose3/1, Matrix Multiply3/5, Matrix Multiply1/4

== system MMMS_v2_dynamics/Dynamic Parameters2/A_connection1 ==
  M0 : Inport
  M0m : Inport  Port=2
  Divide : Product  Inputs=/*  Multiplication=Matrix(*)
  A : Outport
  wires:
  Divide/1 -> A/1
  M0/1 -> Divide/1
  M0m/1 -> Divide/2

== system MMMS_v2_dynamics/Dynamic Parameters2/Mass Matrix Blocks1 ==
  Lm : Inport
  Lm0 : Inport  Port=2
  Xi_m_matrix : Inport  Port=3
  Add : Sum
  Constant1 : Constant  Value=m0_frak  VectorParams1D=off
  Constant2 : Constant  Value=m_diag  VectorParams1D=off
  Matrix Multiply1 : Product  Inputs=4  Multiplication=Matrix(*)
  Matrix Multiply3 : Product  Inputs=5  Multiplication=Matrix(*)
  Matrix Multiply4 : Product  Inputs=3  Multiplication=Matrix(*)
  Matrix Multiply5 : Product  Inputs=1  Multiplication=Matrix(*)
  Transpose3 : Math  Operator=transpose
  Transpose4 : Math  Operator=transpose
  Transpose5 : Math  Operator=transpose
  M0 : Outport
  M0m : Outport  Port=2
  Mm : Outport  Port=3
  wires:
  Xi_m_matrix/1 -> Matrix Multiply1/4, Matrix Multiply3/5, Transpose3/1
  Matrix Multiply5/1 -> M0/1
  Lm0/1 -> Transpose5/1, Matrix Multiply4/3
  Transpose5/1 -> Matrix Multiply4/1, Matrix Multiply1/1
  Transpose4/1 -> Matrix Multiply3/2
  Matrix Multiply3/1 -> Mm/1
  Matrix Multiply1/1 -> M0m/1
  Matrix Multiply4/1 -> Add/2
  Transpose3/1 -> Matrix Multiply3/1
  Lm/1 -> Matrix Multiply1/3, Matrix Multiply3/4, Transpose4/1
  Add/1 -> Matrix Multiply5/1
  Constant2/1 -> Matrix Multiply4/2, Matrix Multiply3/3, Matrix Multiply1/2
  Constant1/1 -> Add/1

== system MMMS_v2_dynamics/Feedback Transformation/Inverse Dynamics1 ==
  note: f_m
  g_I0 : Inport
  "q_m " : Inport  Port=2
  A_dot : MATLAB Function  TreatAsAtomicUnit=on
  Bus Selector : BusSelector  OutputSignals=M0,Mm
  Bus Selector2 : BusSelector  OutputSignals=signal1,signal2
  C_hat : Subsystem  Commented=on
  C_hat1 : Subsystem
  Inverse Dynamics : Subsystem
  M0_dot : MATLAB Function  TreatAsAtomicUnit=on
  N_hat : Subsystem  Commented=on
  N_hat1 : Subsystem
  Scope : Scope
  F_U : Outport
  F_mu : Outport  Port=2
  F_t : Outport  Port=3
  F_m : Outport  Port=4
  N : Outport  Port=5
  tag scope: Chat=global, Nhat=global
  wires:
  [P] -> N_hat1/5(P)
  [Mass_Matrix] -> Bus Selector/1
  Bus Selector/1 -> N_hat1/6(M0), Inverse Dynamics/2(<M0>)  "<M0>"
  g_I0/1 -> N_hat1/1(g_I0), Inverse Dynamics/1(g_I0)
  Inverse Dynamics/1(F_U) -> F_U/1
  Inverse Dynamics/2(F_mu) -> F_mu/1
  Inverse Dynamics/3(F_t) -> F_t/1
  Inverse Dynamics/4(F_m) -> F_m/1
  Bus Selector/2 -> Inverse Dynamics/3(Mm)  "<Mm>"
  Bus Selector2/1 -> C_hat1/1(q_m), N_hat1/2(q_m)  "<signal1>"
  Bus Selector2/2 -> A_dot/2(q_m_dot), M0_dot/2(q_m_dot), C_hat1/2(q_dot_m), N_hat1/3(q_dot_m)  "<signal2>"
  C_hat1/1(M0_partial) -> M0_dot/1(M0_partial)
  C_hat1/2(Out1) -> A_dot/1(A_partial)
  C_hat1/3(C_hat1) -> [Chat], Inverse Dynamics/6(C_hat)
  M0_dot/1(M0_dot) -> Inverse Dynamics/4(M0_dot)
  A_dot/1(A_dot) -> Inverse Dynamics/5(A_dot)
  "q_m "/1 -> Bus Selector2/1
  [A_connection] -> N_hat1/4(A)
  N_hat1/1(N_hat1) -> [Nhat], N/1, Scope/1

== system MMMS_v2_dynamics/Feedback Transformation1/Inverse Dynamics1 ==
  note: f_m
  g_I0 : Inport
  "q_m " : Inport  Port=2
  A_dot : MATLAB Function  TreatAsAtomicUnit=on
  Bus Selector : BusSelector  OutputSignals=M0,Mm
  Bus Selector2 : BusSelector  OutputSignals=signal1,signal2
  C_hat : Subsystem  Commented=on
  C_hat1 : Subsystem
  Inverse Dynamics : Subsystem
  M0_dot : MATLAB Function  TreatAsAtomicUnit=on
  N_hat : Subsystem  Commented=on
  N_hat1 : Subsystem
  Scope : Scope
  F_U : Outport
  F_mu : Outport  Port=2
  F_t : Outport  Port=3
  F_m : Outport  Port=4
  N : Outport  Port=5
  tag scope: Chat2=global, Nhat2=global
  wires:
  [A_connection2] -> N_hat1/4(A)
  "q_m "/1 -> Bus Selector2/1
  A_dot/1(A_dot) -> Inverse Dynamics/5(A_dot)
  M0_dot/1(M0_dot) -> Inverse Dynamics/4(M0_dot)
  C_hat1/2(A_partial) -> A_dot/1(A_partial)
  C_hat1/1(M0_partial1) -> M0_dot/1(M0_partial)
  Bus Selector2/2 -> C_hat1/2(q_dot_m1), N_hat1/3(q_dot_m), M0_dot/2(q_m_dot), A_dot/2(q_m_dot)  "<signal2>"
  Bus Selector2/1 -> C_hat1/1(q_m1), N_hat1/2(q_m)  "<signal1>"
  Bus Selector/2 -> Inverse Dynamics/3(Mm)  "<Mm>"
  Inverse Dynamics/4(F_m) -> F_m/1
  Inverse Dynamics/3(F_t) -> F_t/1
  Inverse Dynamics/2(F_mu) -> F_mu/1
  Inverse Dynamics/1(F_U) -> F_U/1
  g_I0/1 -> Inverse Dynamics/1(g_I0), N_hat1/1(g_I0)
  Bus Selector/1 -> Inverse Dynamics/2(<M0>), N_hat1/6(M0)  "<M0>"
  [Mass_Matrix2] -> Bus Selector/1
  [P2] -> N_hat1/5(P)
  N_hat1/1(N_hat1) -> Scope/1, N/1, [Nhat2]
  C_hat1/3(C_hat3) -> Inverse Dynamics/6(C_hat), [Chat2]

== system MMMS_v2_dynamics/Feedback Transformation2/Inverse Dynamics1 ==
  note: f_m
  g_I0 : Inport
  "q_m " : Inport  Port=2
  A_dot : MATLAB Function  TreatAsAtomicUnit=on
  Bus Selector : BusSelector  OutputSignals=M0,Mm
  Bus Selector2 : BusSelector  OutputSignals=signal1,signal2
  C_hat : Subsystem  Commented=on
  C_hat1 : Subsystem
  Inverse Dynamics : Subsystem
  M0_dot : MATLAB Function  TreatAsAtomicUnit=on
  N_hat : Subsystem  Commented=on
  N_hat1 : Subsystem
  Scope : Scope
  F_U : Outport
  F_mu : Outport  Port=2
  F_t : Outport  Port=3
  F_m : Outport  Port=4
  N : Outport  Port=5
  tag scope: Chat3=global, Nhat3=global
  wires:
  [P3] -> N_hat1/5(P)
  [Mass_Matrix3] -> Bus Selector/1
  Bus Selector/1 -> N_hat1/6(M0), Inverse Dynamics/2(<M0>)  "<M0>"
  g_I0/1 -> N_hat1/1(g_I0), Inverse Dynamics/1(g_I0)
  Inverse Dynamics/1(F_U) -> F_U/1
  Inverse Dynamics/2(F_mu) -> F_mu/1
  Inverse Dynamics/3(F_t) -> F_t/1
  Inverse Dynamics/4(F_m) -> F_m/1
  Bus Selector/2 -> Inverse Dynamics/3(Mm)  "<Mm>"
  Bus Selector2/1 -> C_hat1/1(q_m1), N_hat1/2(q_m)  "<signal1>"
  Bus Selector2/2 -> A_dot/2(q_m_dot), M0_dot/2(q_m_dot), C_hat1/2(q_dot_m1), N_hat1/3(q_dot_m)  "<signal2>"
  C_hat1/1(M0_partial1) -> M0_dot/1(M0_partial)
  C_hat1/2(A_partial) -> A_dot/1(A_partial)
  M0_dot/1(M0_dot) -> Inverse Dynamics/4(M0_dot)
  A_dot/1(A_dot) -> Inverse Dynamics/5(A_dot)
  "q_m "/1 -> Bus Selector2/1
  [A_connection3] -> N_hat1/4(A)
  N_hat1/1(N_hat1) -> N/1, [Nhat3], Scope/1
  C_hat1/3(C_hat3) -> [Chat3], Inverse Dynamics/6(C_hat)

== system MMMS_v2_dynamics/Inverse Dynamics/C_hat ==
  note: C_hat
  q_m1 : Inport
  q_dot_m1 : Inport  Port=2
  A : Inport  Port=3
  <Lm0> : Inport  Port=4
  <Lm> : Inport  Port=5
  <M0> : Inport  Port=6
  <M0m> : Inport  Port=7
  <M0>1 : InportShadow  Port=6
  AMA_partial : MATLAB Function  TreatAsAtomicUnit=on
  A_partial : MATLAB Function  TreatAsAtomicUnit=on
  C_hat1 : MATLAB Function  TreatAsAtomicUnit=on
  Constant : Constant  Value=Xi_m
  Lm_partials : Subsystem
  M_partials : Subsystem
  Mm_hat_partial : MATLAB Function  TreatAsAtomicUnit=on
  M0_partial : Outport
  A_partial1 : Outport  Port=2
  C_hat : Outport  Port=3
  tag scope: A_partial=global, M0_partial=global
  wires:
  M_partials/3(Mm_partial) -> Mm_hat_partial/3(Mm_partial)
  Lm_partials/2(Lm0_partial) -> M_partials/3(Lm0_partial)
  q_m1/1 -> Lm_partials/1(q_m), Mm_hat_partial/1(q_m), C_hat1/1(q_m), AMA_partial/1(q_m), A_partial/1(q_m), M_partials/1(q_m)
  <M0m>/1 -> A_partial/5(M0m)
  Lm_partials/1(Lm_partial) -> M_partials/2(Lm_partial)
  M_partials/1(M0_partial) -> A_partial/3(M0_partial), M0_partial/1, AMA_partial/6(M0_partial), [M0_partial]
  A_partial/1(A_partial) -> AMA_partial/4(A_partial), [A_partial], A_partial1/1
  Constant/1 -> Lm_partials/2(Xi_m)
  M_partials/2(M0m_partial) -> A_partial/4(M0m_partial)
  Mm_hat_partial/1(Mm_hat_partial) -> C_hat1/2(Mm_hat_partial)
  q_dot_m1/1 -> C_hat1/3(q_dot_m)
  AMA_partial/1(AMA_partial) -> Mm_hat_partial/2(AMA_partial)
  <M0>/1 -> A_partial/2(M0)
  [V_I0] -> A_partial/6(V)
  [V_I0] -> M_partials/6(V)
  <Lm>/1 -> M_partials/4(Lm)
  [V_I0] -> AMA_partial/5(V)
  A/1 -> AMA_partial/3(A)
  C_hat1/1(C_hat) -> C_hat/1
  <M0>1/1 -> AMA_partial/2(M0)
  <Lm0>/1 -> M_partials/5(Lm0)

== system MMMS_v2_dynamics/Inverse Dynamics/C_hat1 ==
  q_m : Inport
  q_dot_m : Inport  Port=2
  AMA_partial : MATLAB Function  TreatAsAtomicUnit=on
  A_partial : MATLAB Function  TreatAsAtomicUnit=on
  Bus Selector : BusSelector  OutputSignals=M0,M0m
  Bus Selector1 : BusSelector  OutputSignals=Lm,Lm0
  C_hat : MATLAB Function  TreatAsAtomicUnit=on
  Constant : Constant  Value=Xi_m
  Constant2 : Constant  Commented=on  Value=m_diag  VectorParams1D=off
  Lm_partials : Subsystem
  M_partials : Subsystem
  Mm_hat_partial : MATLAB Function  TreatAsAtomicUnit=on
  M0_partial : Outport
  Out1 : Outport  Port=2
  C_hat1 : Outport  Port=3
  tag scope: A_partial=global, M0_partial=global, Mm_partial=global
  wires:
  [Mass_Matrix] -> Bus Selector/1
  Bus Selector/1 -> AMA_partial/2(M0), A_partial/2(M0)  "<M0>"
  Mm_hat_partial/1(Mm_hat_partial) -> C_hat/2(Mm_hat_partial)
  Constant/1 -> Lm_partials/2(Xi_m)
  q_m/1 -> AMA_partial/1(q_m), C_hat/1(q_m), Mm_hat_partial/1(q_m), A_partial/1(q_m), M_partials/1(q_m), Lm_partials/1(q_m)
  M_partials/3(Mm_partial) -> [Mm_partial], Mm_hat_partial/3(Mm_partial)
  Lm_partials/2(Lm0_partial) -> M_partials/3(Lm0_partial)
  M_partials/2(M0m_partial) -> A_partial/4(M0m_partial)
  AMA_partial/1(AMA_partial) -> Mm_hat_partial/2(AMA_partial)
  Bus Selector1/2 -> M_partials/5(Lm0)  "<Lm0>"
  Lm_partials/1(Lm_partial) -> M_partials/2(Lm_partial)
  A_partial/1(A_partial) -> Out1/1, [A_partial], AMA_partial/4(A_partial)
  C_hat/1(C_hat) -> C_hat1/1
  M_partials/1(M0_partial) -> AMA_partial/6(M0_partial), [M0_partial], M0_partial/1, A_partial/3(M0_partial)
  [V_Ie] -> M_partials/6(V)
  Bus Selector/2 -> A_partial/5(M0m)  "<M0m>"
  q_dot_m/1 -> C_hat/3(q_dot_m)
  [V_Ie] -> A_partial/6(V)
  [V_Ie] -> AMA_partial/5(V)
  [A_connection] -> AMA_partial/3(A)
  [L] -> Bus Selector1/1
  Bus Selector1/1 -> M_partials/4(Lm)  "<Lm>"

== system MMMS_v2_dynamics/Inverse Dynamics/Inverse Dynamics ==
  note: Subsystem
  note: Inverse dynamics
  g_I0 : Inport
  <M0> : Inport  Port=2
  Mm : Inport  Port=3
  M0_dot : Inport  Port=4
  A_dot : Inport  Port=5
  C_hat : Inport  Port=6
  <M0>2 : InportShadow  Port=2
  Ad_g_I0_dot : MATLAB Function  TreatAsAtomicUnit=on
  Ad_g_I0_dot1 : MATLAB Function  TreatAsAtomicUnit=on
  Ad_g_te_dot : MATLAB Function  TreatAsAtomicUnit=on
  FU : MATLAB Function  TreatAsAtomicUnit=on
  Fm : MATLAB Function  TreatAsAtomicUnit=on
  Fmu : MATLAB Function  TreatAsAtomicUnit=on
  Gain : Gain  Commented=on  Gain=-1
  Goto : Goto  Commented=on  GotoTag=JJ  TagVisibility=global
  Inverse Dynamics : MATLAB Function  Commented=on  TreatAsAtomicUnit=on
  MATLAB Function3 : MATLAB Function  TreatAsAtomicUnit=on
  MmJcross : MATLAB Function  TreatAsAtomicUnit=on
  Mm_hat : MATLAB Function  TreatAsAtomicUnit=on
  Mt : Constant  Value=M_t
  Scope1 : Scope
  Scope2 : Scope
  F_U : Outport
  F_mu : Outport  Port=2
  F_t : Outport  Port=3
  F_m : Outport  Port=4
  wires:
  Mm/1 -> Mm_hat/2(Mm)
  [A_connection] -> Mm_hat/3(A), MmJcross/2(A)
  FU/1(F_U) -> F_U/1
  Fmu/1(F_mu) -> F_mu/1
  MATLAB Function3/1(F_t) -> F_t/1
  Fm/1(F_m) -> F_m/1
  <M0>/1 -> Mm_hat/1(M0)
  C_hat/1 -> Fm/3(Cm_hat)
  <M0>2/1 -> Fmu/2(M0)
  g_I0/1 -> Fmu/4(g_I0), Ad_g_I0_dot/1(g_I0)
  M0_dot/1 -> Fmu/3(M_0_dot)
  A_dot/1 -> Fm/2(A_dot)
  [V_Ie] -> Ad_g_I0_dot/2(V_I0)
  Ad_g_I0_dot1/1(Ad_g_It_dot) -> MATLAB Function3/6(Ad_gIt_dot)
  Ad_g_I0_dot/1(Ad_g_I0_dot) -> Fmu/5(Ad_g_I0_dot)
  Ad_g_te_dot/1(Ad_g_te_dot) -> MATLAB Function3/5(Ad_gte_dot)
  [g_te] -> MATLAB Function3/2(g_te), Ad_g_te_dot/2(g_te)
  [g_It] -> MATLAB Function3/3(g_It), Ad_g_I0_dot1/2(g_It)
  [V_te] -> Ad_g_te_dot/1(V_te)
  [V_It] -> Ad_g_I0_dot1/1(V_t)
  Mt/1 -> MATLAB Function3/4(Mt)
  Mm_hat/1(Mm_hat) -> MmJcross/1(Mm_hat), Scope1/1
  MmJcross/1(MmJcross) -> FU/1(MmJcross), MATLAB Function3/1(MmJcross), Fmu/1(MmJcross), Fm/1(MmJcross), Scope2/1
  Gain/1 -> Goto/1

== system MMMS_v2_dynamics/Inverse Dynamics/N_hat ==
  q_m : Inport
  q_dot_m : Inport  Port=2
  A : Inport  Port=3
  P : Inport  Port=4
  M0 : Inport  Port=5
  Constant : Constant  Value=iota0
  Matrix Multiply : Product  Multiplication=Matrix(*)
  N_hat : MATLAB Function  TreatAsAtomicUnit=on
  To Workspace : ToWorkspace  VariableName=N_firstpart  SaveFormat=Timeseries  SampleTime=-1
  N_hat1 : Outport
  wires:
  P/1 -> Matrix Multiply/2, N_hat/5(P)
  [M0_partial] -> N_hat/6(M0_partial)
  N_hat/1(N_hat_temp) -> To Workspace/1, Matrix Multiply/1
  q_m/1 -> N_hat/1(q_m)
  q_dot_m/1 -> N_hat/2(q_dot_m)
  [V_I0] -> N_hat/4(V)
  A/1 -> N_hat/3(A)
  [A_partial] -> N_hat/7(A_partial)
  Constant/1 -> N_hat/8(iota0)
  Matrix Multiply/1 -> N_hat1/1
  M0/1 -> N_hat/9(M0)
